simulink model "Cascade_FIR_Ref"  (R2020b)
settings: Solver=FixedStepAuto  StartTime=0.0  StopTime=10.0  FixedStep=0.1  RelTol=1e-3
settings Model: Creator=Shubham  LastModifiedBy=Shubham
settings DataIOCC: SaveOutput=off  SaveTime=off

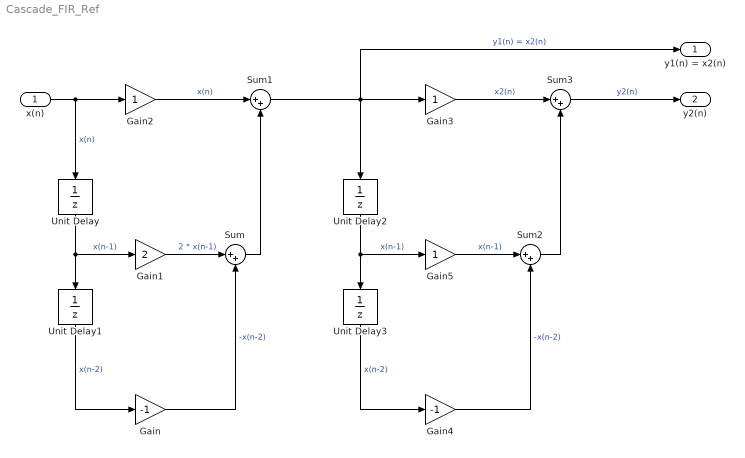
== system Cascade_FIR_Ref ==
  x(n) : Inport  OutDataTypeStr=double  PortDimensions=1  SampleTime=[0.10000000000000001,0]
  Gain : Gain  Gain=-1
  Gain1 : Gain  Gain=2
  Gain2 : Gain
  Gain3 : Gain
  Gain4 : Gain  Gain=-1
  Gain5 : Gain
  Sum{,1..3} (4 alike) : Sum  Inputs=|++
  Unit Delay{,1..3} (4 alike) : UnitDelay  SampleTime=-1  HasFrameUpgradeWarning=on
  y1(n) = x2(n) : Outport  OutDataTypeStr=double  PortDimensions=1  SampleTime=[0.10000000000000001,0]
  y2(n) : Outport  Port=2  OutDataTypeStr=double  PortDimensions=1  SampleTime=[0.10000000000000001,0]
  wires:
  Sum/1 -> Sum1/2
  Unit Delay/1 -> Gain1/1, Unit Delay1/1  "x(n-1)"
  Sum1/1 -> Gain3/1, Unit Delay2/1, y1(n) = x2(n)/1  "y1(n) = x2(n)"
  Gain1/1 -> Sum/1  "2 * x(n-1)"
  Gain4/1 -> Sum2/2  "-x(n-2)"
  Gain/1 -> Sum/2  "-x(n-2)"
  Unit Delay1/1 -> Gain/1  "x(n-2)"
  Gain5/1 -> Sum2/1  "x(n-1)"
  Gain2/1 -> Sum1/1  "x(n)"
  Unit Delay2/1 -> Unit Delay3/1, Gain5/1  "x(n-1)"
  x(n)/1 -> Unit Delay/1, Gain2/1  "x(n)"
  Gain3/1 -> Sum3/1  "x2(n)"
  Unit Delay3/1 -> Gain4/1  "x(n-2)"
  Sum2/1 -> Sum3/2
  Sum3/1 -> y2(n)/1  "y2(n)"
